simulink model "powerwindow03"  (R2019b)
settings: Solver=ode23tb  StartTime=0.0  StopTime=inf  FixedStep=1e-4  RelTol=1e-2  EnableMultiTasking=on
libraries: mblibv1 x19, powerlib x15, simulink x4, vrlib x1
(part 1 of 2)
settings Model: FPTRunName=Active  ExtModeAutoUpdateStatusClock=off  Creator=The MathWorks Inc.  LastModifiedBy=bhisma
settings DataIOCC: LimitDataPoints=on  SaveFormat=Array  SignalLoggingSaveFormat=ModelDataLogs  ReturnWorkspaceOutputs=off  SignalLoggingName=sigsOut
settings OptimizationCC: BooleanDataType=off  ExpressionDepthLimit=2147483647  InitFltsAndDblsToZero=on  LifeSpan=inf
settings DebuggingCC: SaveWithParameterizedLinksMsg=none  UnderspecifiedInitializationDetection=Classic  MergeDetectMultiDrivingBlocksExec=none  CheckExecutionContextPreStartOutputMsg=on  CheckExecutionContextRuntimeOutputMsg=on  SignalResolutionControl=TryResolveAllWithWarning  MultiTaskDSMMsg=warning  MultiTaskCondExecSysMsg=none  FcnCallInpInsideContextMsg=warning  StateNameClashWarn=warning  SFUnexpectedBacktrackingDiag=warning  SFNoUnconditionalDefaultTransitionDiag=warning  SFExecutionAtInitializationDiag=none  ArithmeticOperatorsInVariantConditions=warning
settings HardwareCC: ProdBitPerPointer=32  ProdBitPerSizeT=32  ProdBitPerPtrDiffT=32  ProdLargestAtomicFloat=None  ProdIntDivRoundTo=Undefined  ProdEndianess=Unspecified  ProdWordSize=32  ProdHWDeviceType=32-bit Generic
settings ModelReferenceCC: PropagateSignalLabelsOutOfModel=off
settings SFSimCC: SimUseLocalCustomCode=off  SimParseCustomCode=off  CustomCodeUndefinedFunction=UseInterfaceOnly
settings RTWCC: RTWUseLocalCustomCode=off
settings CodeAppCC: StateflowObjectComments=on
settings GRTTargetCC: TargetFcnLib=ansi_tfl_tmw.mat  TargetLangStandard=C89/C90 (ANSI)  GeneratePreprocessorConditionals=Disable all  CombineOutputUpdateFcns=off  GRTInterface=on
settings ConfigComp: CovMetricSettings=dw  CovHtmlReporting=on  CovSaveCumulativeToWorkspaceVar=on  CovSaveSingleToWorkspaceVar=on  CovExternalEMLEnable=off
settings SimscapeCC: SimscapeNormalizeSystem=off
settings SimMechanicsCC: WarnOnRedundantConstraints=off  VisOnUpdateDiagram=on

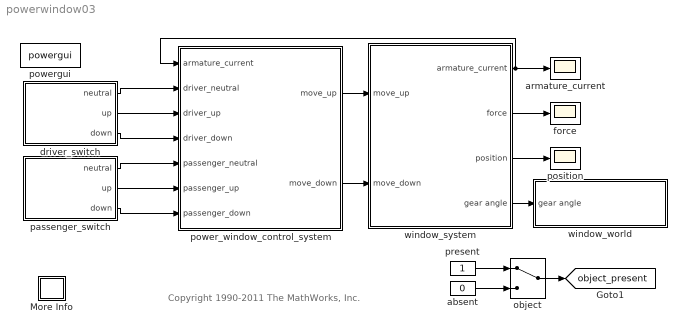
== system powerwindow03 ==
  note: Copyright 1990-2011 The MathWorks, Inc.
  More Info : Subsystem
      settings: OpenFcn=showdemo(bdroot(gcb))
      mask Display: disp('?')
  absent : Constant  Value=0
  armature_current : Scope
  driver_switch : Subsystem
  force : Scope
  object : ManualSwitch
  passenger_switch : Subsystem
  position : Scope
  power_window_control_system : Subsystem
  powergui : powerlib/powergui  SimulationMode=Continuous  SampleTime=0  frequency=60  Iterations=50  frequencyindice=0  Pbase=100e6  ErrMax=1e-4  UnitsV=kV  UnitsW=MW  buscounter=0  FunctionMessages=off  echomessages=off  EnableUseOfTLC=off  CurrentSourceSwitches=off  DisableSnubberDevices=off  DisableRonSwitches=off  DisableVfSwitches=off  DisplayEquations=off  AutomaticDiscreteSolvers=off  SolverType=Tustin  Interpol=off  ExternalGateDelay=off  methode=off  Ts=0  x0status=blocks  SPID=off  SwTol=0  HookPort=off  NonlinearTolerance=1e-4  nMaxIteration=100  ContinueOnMaxIteration=off  RestoreLinks=warning  ResistiveCurrentMeasurement=off  Frange=[0:2:500]  Ylog=off  Xlog=on  ShowGrid=off  save=off  variable=ZData  structure=0  ZoomFFT=on  StartTime=0.0  cycles=1  DisplayStyle=1  fundamental=60  FreqAxis=off  MaxFrequency=1000  frequencyindicesteady=1  RmsSteady=1  display=off
      settings: SourceProductName=Simscape Electrical
  present : Constant
  window_system : Subsystem
  window_world : Subsystem
  tag scope: object_present=global
  wires:
  driver_switch/1(neutral) -> power_window_control_system/2(driver_neutral)
  driver_switch/2(up) -> power_window_control_system/3(driver_up)
  driver_switch/3(down) -> power_window_control_system/4(driver_down)
  passenger_switch/1(neutral) -> power_window_control_system/5(passenger_neutral)
  passenger_switch/2(up) -> power_window_control_system/6(passenger_up)
  passenger_switch/3(down) -> power_window_control_system/7(passenger_down)
  power_window_control_system/1(move_up) -> window_system/1(move_up)
  power_window_control_system/2(move_down) -> window_system/2(move_down)
  window_system/1(armature_current) -> armature_current/1, power_window_control_system/1(armature_current)
  window_system/2(force) -> force/1
  window_system/3(position) -> position/1
  present/1 -> object/1
  absent/1 -> object/2
  object/1 -> [object_present]
  window_system/4(gear angle) -> window_world/1(gear angle)

== system powerwindow03/More Info ==

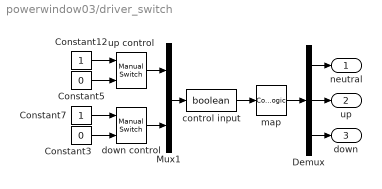
== system powerwindow03/driver_switch ==
  Constant12 : Constant
  Constant3 : Constant  Value=0
  Constant5 : Constant  Value=0
  Constant7 : Constant
  Demux : Demux  Outputs=3
  Mux1 : Mux  Inputs=2
  control input : DataTypeConversion  OutDataTypeStr=boolean  SaturateOnIntegerOverflow=on  RndMeth=Zero
  down control : simulink/Signal Routing/Manual Switch  sw=0  action=0  varsize=off
      settings: SourceProductName=Simulink  SourceProductBaseCode=SL
  map : CombinatorialLogic  TruthTable=[1 0 0;0 0 1;0 1 0;1 0 0]
  up control : simulink/Signal Routing/Manual Switch  sw=1  action=0  varsize=off
      settings: SourceProductName=Simulink  SourceProductBaseCode=SL
  neutral : Outport
  up : Outport  Port=2
  down : Outport  Port=3
  wires:
  control input/1 -> map/1
  Constant12/1 -> up control/1
  Constant5/1 -> up control/2
  Constant7/1 -> down control/1
  Constant3/1 -> down control/2
  down control/1 -> Mux1/2
  Mux1/1 -> control input/1
  up control/1 -> Mux1/1
  map/1 -> Demux/1
  Demux/1 -> neutral/1
  Demux/2 -> up/1
  Demux/3 -> down/1

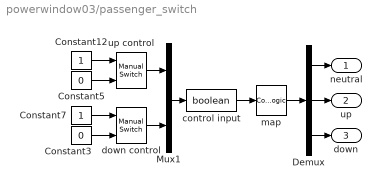
== system powerwindow03/passenger_switch ==
  Constant12 : Constant
  Constant3 : Constant  Value=0
  Constant5 : Constant  Value=0
  Constant7 : Constant
  Demux : Demux  Outputs=3
  Mux1 : Mux  Inputs=2
  control input : DataTypeConversion  OutDataTypeStr=boolean  SaturateOnIntegerOverflow=on  RndMeth=Zero
  down control : simulink/Signal Routing/Manual Switch  sw=0  action=0  varsize=off
      settings: SourceProductName=Simulink  SourceProductBaseCode=SL
  map : CombinatorialLogic  TruthTable=[1 0 0;0 0 1;0 1 0;1 0 0]
  up control : simulink/Signal Routing/Manual Switch  sw=0  action=0  varsize=off
      settings: SourceProductName=Simulink  SourceProductBaseCode=SL
  neutral : Outport
  up : Outport  Port=2
  down : Outport  Port=3
  wires:
  Demux/3 -> down/1
  Demux/2 -> up/1
  Demux/1 -> neutral/1
  map/1 -> Demux/1
  up control/1 -> Mux1/1
  Mux1/1 -> control input/1
  down control/1 -> Mux1/2
  Constant3/1 -> down control/2
  Constant7/1 -> down control/1
  Constant5/1 -> up control/2
  Constant12/1 -> up control/1
  control input/1 -> map/1

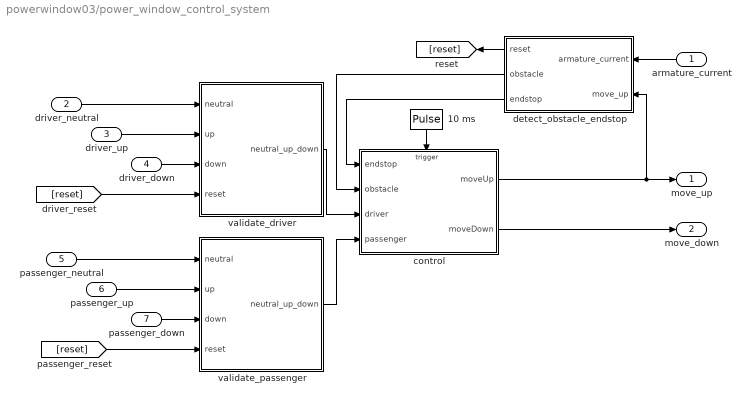
== system powerwindow03/power_window_control_system ==
  armature_current : Inport
  driver_neutral : Inport  Port=2
  driver_up : Inport  Port=3
  driver_down : Inport  Port=4
  passenger_neutral : Inport  Port=5
  passenger_up : Inport  Port=6
  passenger_down : Inport  Port=7
  10 ms : DiscretePulseGenerator  SampleTime=10e-3
  control : Stateflow chart  TreatAsAtomicUnit=on
  detect_obstacle_endstop : Subsystem
  validate_driver : Subsystem
  validate_passenger : Subsystem
  move_up : Outport
  move_down : Outport  Port=2
  wires:
  detect_obstacle_endstop/2(obstacle) -> control/2(obstacle)
  detect_obstacle_endstop/3(endstop) -> control/1(endstop)
  detect_obstacle_endstop/1(reset) -> [reset]
  armature_current/1 -> detect_obstacle_endstop/1(armature_current)
  10 ms/1 -> control/Trigger
  control/1(moveUp) -> detect_obstacle_endstop/2(move_up), move_up/1
  control/2(moveDown) -> move_down/1
  driver_neutral/1 -> validate_driver/1(neutral)
  driver_up/1 -> validate_driver/2(up)
  driver_down/1 -> validate_driver/3(down)
  [reset] -> validate_driver/4(reset)
  passenger_neutral/1 -> validate_passenger/1(neutral)
  passenger_up/1 -> validate_passenger/2(up)
  passenger_down/1 -> validate_passenger/3(down)
  [reset] -> validate_passenger/4(reset)
  validate_driver/1(neutral_up_down) -> control/3(driver)
  validate_passenger/1(neutral_up_down) -> control/4(passenger)

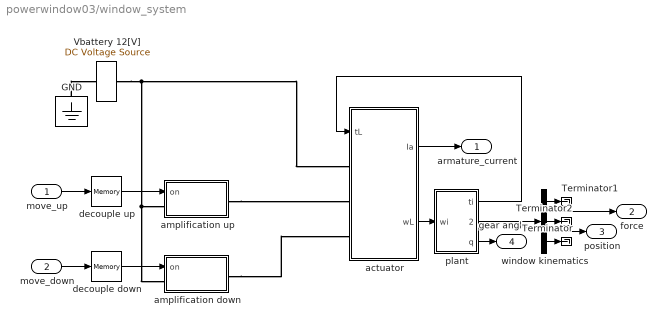
== system powerwindow03/window_system ==
  move_up : Inport
  move_down : Inport  Port=2
  GND : powerlib/Elements/Ground  LConnTagsString=a
      settings: SourceProductName=Simscape Electrical
  Terminator : Terminator
  Terminator1 : Terminator
  Terminator2 : Terminator
  Vbattery 12[V] : powerlib/Electrical Sources/DC Voltage Source  Amplitude=12  Measurements=None
      settings: SourceProductName=Simscape Electrical
  actuator : Subsystem
  amplification down : Subsystem
  amplification up : Subsystem
  decouple down : Memory
  decouple up : Memory
  plant : Subsystem
  window kinematics : Demux  Outputs=[1,1,2,1,4]
  armature_current : Outport
  force : Outport  Port=2
  position : Outport  Port=3
  gear angle : Outport  Port=4
  wires:
  decouple down/1 -> amplification down/1(on)
  decouple up/1 -> amplification up/1(on)
  plant/3(q) -> gear angle/1
  actuator/2(wL) -> plant/1(wi)
  plant/2("F, x, v") -> window kinematics/1
  actuator/1(Ia) -> armature_current/1
  move_up/1 -> decouple up/1
  move_down/1 -> decouple down/1
  window kinematics/2 -> force/1
  window kinematics/1 -> Terminator1/1
  window kinematics/4 -> position/1
  window kinematics/5 -> Terminator/1
  window kinematics/3 -> Terminator2/1
  plant/1(ti) -> actuator/1(tL)
  connections:
  GND/LConn1 -- Vbattery 12[V]/LConn1
  amplification up/RConn1 -- actuator/LConn2
  amplification down/RConn1 -- actuator/LConn3
  Vbattery 12[V]/RConn1 -- amplification down/LConn1 -- amplification up/LConn1 -- actuator/LConn1

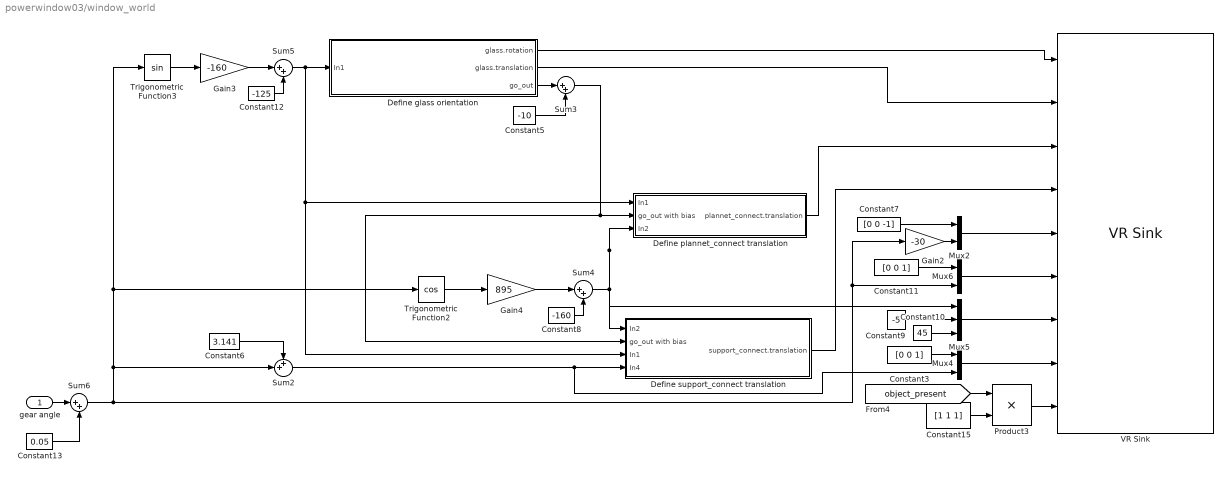
== system powerwindow03/window_world ==
  gear angle : Inport
  Constant10 : Constant  Value=45
  Constant11 : Constant  Value=[0 0 1]
  Constant12 : Constant  Value=-125
  Constant13 : Constant  Value=0.05
  Constant15 : Constant  Value=[1 1 1]
  Constant3 : Constant  Value=[0 0 1]
  Constant5 : Constant  Value=-10
  Constant6 : Constant  Value=3.141
  Constant7 : Constant  Value=[0 0 -1]
  Constant8 : Constant  Value=-160
  Constant9 : Constant  Value=-5
  Define glass orientation : Subsystem
  Define plannet_connect translation : Subsystem
  Define support_connect translation : Subsystem
  Gain2 : Gain  Gain=-30  SaturateOnIntegerOverflow=on  OutDataTypeStr=Inherit: Same as input  ParamDataTypeStr=Inherit: Same as input
  Gain3 : Gain  Gain=-160  SaturateOnIntegerOverflow=on  OutDataTypeStr=Inherit: Same as input  ParamDataTypeStr=Inherit: Same as input
  Gain4 : Gain  Gain=895  SaturateOnIntegerOverflow=on  OutDataTypeStr=Inherit: Same as input  ParamDataTypeStr=Inherit: Same as input
  Mux2 : Mux  Inputs=2
  Mux4 : Mux  Inputs=2
  Mux5 : Mux  Inputs=3
  Mux6 : Mux  Inputs=2
  Product3 : Product  SaturateOnIntegerOverflow=on  InputSameDT=on  OutDataTypeStr=Inherit: Same as first input
  Sum2 : Sum  Inputs=++|  SaturateOnIntegerOverflow=on  InputSameDT=on  OutDataTypeStr=Inherit: Same as first input
  Sum{3..6} (4 alike) : Sum  Inputs=|++  SaturateOnIntegerOverflow=on  InputSameDT=on  OutDataTypeStr=Inherit: Same as first input
  Trigonometric Function2 : Trigonometry  Operator=cos
  Trigonometric Function3 : Trigonometry
  VR Sink : vrlib/VR Sink  SampleTime=0.1  ViewEnable=on  RemoteChange=off  RemoteView=on  FieldsWritten=glass.rotation.4.1.1.double#glass.translation.3.1.1.double#plannet_connect.translation.3.1.1.double#support_connect.translation.3.1.1.double#worm.rotation.4.1.1.double#planetROT.rotation.4.1.1.double#support.translation.3.1.1.double#supportROT.rotation.4.1.1.double#balloon.scale.3.1.1.double  WorldFileName=pw_mech_window_world.wrl  WorldDescription=VR Power Window Model  AutoView=on  VideoDimensions=[]  AllowVariableSize=off  FigureProperties="{'Position', 'Name', 'Viewpoint', 'CameraBound', 'CameraDirection', 'CameraPosition', 'CameraUpVector', 'ZoomFactor', 'Antialiasing', 'Headlight', 'Lighting', 'NavPanel', 'StatusBar', 'ToolBar', 'Textures', 'Transparency', 'Wireframe', 'NavZones', 'NavMode', 'NavSpeed', 'Record2DCompressMethod', 'Record2DCompressQuality', 'Record2D', 'Record2DFileName', 'Record2DFPS'; [3.3000000000000000e+01   5.5200000000000000e+02   5.7600000000000000e+02   3.8000000000000000e+02], 'VR Power Window Model', 'Main View', 'on', [0.0000000000000000e+00   0.0000000000000000e+00  -1.0000000000000000e+00], [0.0000000000000000e+00   0.0000000000000000e+00   0.0000000000000000e+00], [0.0000000000000000e+00   1.0000000000000000e+00   0.0000000000000000e+00], [1.0000000000000000e+00], 'off', 'on', 'on', 'halfbar', 'on', 'on', 'on', 'on', 'off', 'off', 'examine', 'normal', 'auto', [7.5000000000000000e+01], 'off', '%f_anim_%n.avi', [1.5000000000000000e+01]}"
      settings: SourceProductName=Simulink
  wires:
  Constant5/1 -> Sum3/2
  Constant7/1 -> Mux2/1
  Gain2/1 -> Mux2/2
  Gain3/1 -> Sum5/1
  Constant12/1 -> Sum5/2
  Constant11/1 -> Mux6/1
  Trigonometric Function3/1 -> Gain3/1
  Constant8/1 -> Sum4/2
  Gain4/1 -> Sum4/1
  Trigonometric Function2/1 -> Gain4/1
  Constant10/1 -> Mux5/3
  Constant9/1 -> Mux5/2
  Sum2/1 -> Define support_connect translation/4(In4), Mux4/2
  Constant3/1 -> Mux4/1
  gear angle/1 -> Sum6/1
  Constant13/1 -> Sum6/2
  Constant15/1 -> Product3/2
  [object_present] -> Product3/1
  Define glass orientation/3(go_out) -> Sum3/1
  Sum6/1 -> Mux6/2, Gain2/1, Sum2/2, Trigonometric Function3/1, Trigonometric Function2/1
  Sum3/1 -> Define support_connect translation/2(go_out with bias), Define plannet_connect translation/2(go_out with bias)
  Sum5/1 -> Define plannet_connect translation/1(In1), Define support_connect translation/3(In1), Define glass orientation/1(In1)
  Sum4/1 -> Mux5/1, Define plannet_connect translation/3(In2), Define support_connect translation/1(In2)
  Constant6/1 -> Sum2/1
  Define glass orientation/1(glass.rotation) -> VR Sink/1
  Define glass orientation/2(glass.translation) -> VR Sink/2
  Define plannet_connect translation/1(plannet_connect.translation) -> VR Sink/3
  Mux2/1 -> VR Sink/5
  Mux6/1 -> VR Sink/6
  Mux5/1 -> VR Sink/7
  Define support_connect translation/1(support_connect.translation) -> VR Sink/4
  Mux4/1 -> VR Sink/8
  Product3/1 -> VR Sink/9

== system powerwindow03/power_window_control_system/detect_obstacle_endstop ==
  armature_current : Inport
  move_up : Inport  Port=2
  detect_endstop : Subsystem
  detect_obstacle : Subsystem
  either : Logic  Operator=OR
  process_current : Subsystem
  reset : Outport
  obstacle : Outport  Port=2
  endstop : Outport  Port=3
  wires:
  armature_current/1 -> process_current/1(raw_current)
  detect_obstacle/1(obstacle) -> either/1, obstacle/1
  detect_endstop/1(endstop) -> endstop/1, either/2
  either/1 -> reset/1
  move_up/1 -> detect_obstacle/1(move_up)
  process_current/1(processed_current) -> detect_obstacle/2(armature_current), detect_endstop/1(armature_current)

== system powerwindow03/power_window_control_system/validate_driver ==
  neutral : Inport
  up : Inport  Port=2
  down : Inport  Port=3
  reset : Inport  Port=4
  Mux : Mux  Inputs=3
  check_down : Subsystem
  check_up : Subsystem
  mutually_exclusive : Subsystem
  neutral_up_down : Outport
  wires:
  Mux/1 -> neutral_up_down/1
  reset/1 -> [reset]
  [reset] -> check_down/2(reset)
  [reset] -> check_up/2(reset)
  check_up/1(checked_action) -> mutually_exclusive/2(up)
  neutral/1 -> mutually_exclusive/1(neutral)
  up/1 -> check_up/1(action)
  down/1 -> check_down/1(action)
  mutually_exclusive/1(validated_neutral) -> Mux/1
  mutually_exclusive/2(validated_up) -> Mux/2
  mutually_exclusive/3(validated_down) -> Mux/3
  check_down/1(checked_action) -> mutually_exclusive/3(down)

== system powerwindow03/power_window_control_system/validate_passenger ==
  neutral : Inport
  up : Inport  Port=2
  down : Inport  Port=3
  reset : Inport  Port=4
  Mux : Mux  Inputs=3
  check_down : Subsystem
  check_up : Subsystem
  mutually_exclusive : Subsystem
  neutral_up_down : Outport
  wires:
  Mux/1 -> neutral_up_down/1
  reset/1 -> [reset]
  [reset] -> check_down/2(reset)
  [reset] -> check_up/2(reset)
  check_up/1(checked_action) -> mutually_exclusive/2(up)
  neutral/1 -> mutually_exclusive/1(neutral)
  up/1 -> check_up/1(action)
  down/1 -> check_down/1(action)
  mutually_exclusive/1(validated_neutral) -> Mux/1
  mutually_exclusive/2(validated_up) -> Mux/2
  mutually_exclusive/3(validated_down) -> Mux/3
  check_down/1(checked_action) -> mutually_exclusive/3(down)

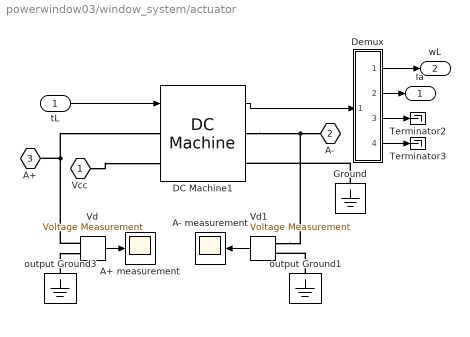
== system powerwindow03/window_system/actuator ==
  tL : Inport
  A+ measurement : Scope
  A- measurement : Scope
  DC Machine1 : powerlib/Machines/DC Machine  PresetModel=No  MechanicalLoad=Torque TL  FieldType=Wound  ShowDetailedParameters=on  RLa="[0.15  0.036]"  RLf=[1.5 3]  Laf=1  MachineConstant=Torque constant (N.m/A)  Ke=1.8  Kt=1.8  J=0.085  Bm=5  Tf=0  w0=0  Ifinit=8  TsPowergui=0  TsBlock=-1
      settings: SourceProductName=Simscape Electrical
  Demux : Subsystem
  Ground : powerlib/Elements/Ground  LConnTagsString=a
      settings: SourceProductName=Simscape Electrical
  Terminator2 : Terminator
  Terminator3 : Terminator
  Vd : powerlib/Measurements/Voltage Measurement  PhasorSimulation=off  OutputType=Magnitude  PSBequivalent=0
      settings: SourceProductName=Simscape Electrical
  Vd1 : powerlib/Measurements/Voltage Measurement  PhasorSimulation=off  OutputType=Magnitude  PSBequivalent=0
      settings: SourceProductName=Simscape Electrical
  output Ground1 : powerlib/Elements/Ground  LConnTagsString=a
      settings: SourceProductName=Simscape Electrical
  output Ground3 : powerlib/Elements/Ground  LConnTagsString=a
      settings: SourceProductName=Simscape Electrical
  Vcc : PMIOPort  Side=Left
  A- : PMIOPort  Port=2  Side=Left
  A+ : PMIOPort  Port=3  Side=Left
  Ia : Outport
  wL : Outport  Port=2
  wires:
  Demux/4(Te) -> Terminator3/1
  Demux/3(If) -> Terminator2/1
  DC Machine1/1 -> Demux/1(m)
  Demux/2(Ia) -> Ia/1
  Vd/1 -> A+ measurement/1
  Vd1/1 -> A- measurement/1
  Demux/1(wm) -> wL/1
  tL/1 -> DC Machine1/1
  connections:
  output Ground3/LConn1 -- Vd/LConn2
  output Ground1/LConn1 -- Vd1/LConn2
  Ground/LConn1 -- DC Machine1/RConn2
  Vd1/LConn1 -- A-/RConn1 -- DC Machine1/RConn1
  Vcc/RConn1 -- DC Machine1/LConn2
  Vd/LConn1 -- A+/RConn1 -- DC Machine1/LConn1

== system powerwindow03/window_system/amplification down ==
  on : Inport
  Logical Operator : Logic  Operator=NOT
  Terminator1 : Terminator
  Terminator2 : Terminator
  output Ground1 : powerlib/Elements/Ground  LConnTagsString=a
      settings: SourceProductName=Simscape Electrical
  up switch : powerlib/Power Electronics/Ideal Switch  Ron=0.01  Lon=0  IC=0  Rs=1000000  Cs=inf  Measurements=on
      settings: SourceProductName=Simscape Electrical
  up switch1 : powerlib/Power Electronics/Ideal Switch  Ron=0.01  Lon=0  IC=0  Rs=1000000  Cs=inf  Measurements=on
      settings: SourceProductName=Simscape Electrical
  Vcc : PMIOPort  Side=Left
  pin : PMIOPort  Port=2  Side=Right
  wires:
  on/1 -> up switch/1, Logical Operator/1
  up switch/1 -> Terminator1/1
  up switch1/1 -> Terminator2/1
  Logical Operator/1 -> up switch1/1
  connections:
  Vcc/RConn1 -- up switch/LConn1
  up switch/RConn1 -- pin/RConn1 -- up switch1/RConn1
  up switch1/LConn1 -- output Ground1/LConn1

== system powerwindow03/window_system/amplification up ==
  on : Inport
  Logical Operator : Logic  Operator=NOT
  Terminator1 : Terminator
  Terminator2 : Terminator
  output Ground1 : powerlib/Elements/Ground  LConnTagsString=a
      settings: SourceProductName=Simscape Electrical
  up switch : powerlib/Power Electronics/Ideal Switch  Ron=0.01  Lon=0  IC=0  Rs=1000000  Cs=inf  Measurements=on
      settings: SourceProductName=Simscape Electrical
  up switch1 : powerlib/Power Electronics/Ideal Switch  Ron=0.01  Lon=0  IC=0  Rs=1000000  Cs=inf  Measurements=on
      settings: SourceProductName=Simscape Electrical
  Vcc : PMIOPort  Side=Left
  pin : PMIOPort  Port=2  Side=Right
  wires:
  on/1 -> up switch/1, Logical Operator/1
  up switch/1 -> Terminator1/1
  up switch1/1 -> Terminator2/1
  Logical Operator/1 -> up switch1/1
  connections:
  Vcc/RConn1 -- up switch/LConn1
  up switch1/LConn1 -- output Ground1/LConn1
  pin/RConn1 -- up switch/RConn1 -- up switch1/RConn1

== system powerwindow03/window_system/plant ==
  wi : Inport
  Demux1 : Demux  Outputs=[4, 1, 2, 1, 1]
  Terminator : Terminator
  Terminator1 : Terminator
  Terminator2 : Terminator
  object : Subsystem
  window : Subsystem
  ti : Outport
  "F, x, v" : Outport  Port=2
  q : Outport  Port=3
  wires:
  window/2(ti) -> ti/1
  wi/1 -> window/1(wi)
  object/1(torque) -> window/2(Fx)
  window/3(q) -> q/1
  Demux1/4 -> object/2(velocity)
  Demux1/2 -> object/1(position)
  Demux1/1 -> Terminator/1
  Demux1/3 -> Terminator1/1
  Demux1/5 -> Terminator2/1
  window/1(F,d,v) -> Demux1/1, "F, x, v"/1

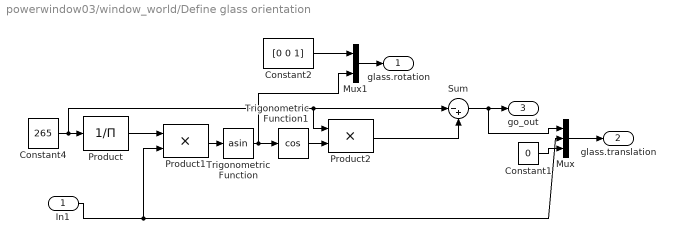
== system powerwindow03/window_world/Define glass orientation ==
  In1 : Inport
  Constant1 : Constant  Value=0
  Constant2 : Constant  Value=[0 0 1]
  Constant4 : Constant  Value=265
  Mux : Mux  Inputs=3
  Mux1 : Mux  Inputs=2
  Product : Product  Inputs=/  SaturateOnIntegerOverflow=on  InputSameDT=on  OutDataTypeStr=Inherit: Same as first input
  Product1 : Product  SaturateOnIntegerOverflow=on  InputSameDT=on  OutDataTypeStr=Inherit: Same as first input
  Product2 : Product  SaturateOnIntegerOverflow=on  InputSameDT=on  OutDataTypeStr=Inherit: Same as first input
  Sum : Sum  Inputs=|-+  SaturateOnIntegerOverflow=on  InputSameDT=on  OutDataTypeStr=Inherit: Same as first input
  Trigonometric Function : Trigonometry  Operator=asin
  Trigonometric Function1 : Trigonometry  Operator=cos
  glass.rotation : Outport
  glass.translation : Outport  Port=2
  go_out : Outport  Port=3
  wires:
  Mux/1 -> glass.translation/1
  Mux1/1 -> glass.rotation/1
  In1/1 -> Product1/2, Mux/2
  Constant1/1 -> Mux/3
  Constant2/1 -> Mux1/1
  Constant4/1 -> Product/1, Product2/1, Sum/1
  Product/1 -> Product1/1
  Product1/1 -> Trigonometric Function/1
  Trigonometric Function/1 -> Trigonometric Function1/1, Mux1/2
  Trigonometric Function1/1 -> Product2/2
  Product2/1 -> Sum/2
  Sum/1 -> go_out/1, Mux/1

== system powerwindow03/window_world/Define plannet_connect translation ==
  In1 : Inport
  go_out with bias : Inport  Port=2
  In2 : Inport  Port=3
  Gain1 : Gain  Gain=0.265  SaturateOnIntegerOverflow=on  OutDataTypeStr=Inherit: Same as input  ParamDataTypeStr=Inherit: Same as input
  Mux3 : Mux  Inputs=3
  plannet_connect.translation : Outport
  wires:
  Mux3/1 -> plannet_connect.translation/1
  In2/1 -> Gain1/1
  In1/1 -> Mux3/2
  go_out with bias/1 -> Mux3/1
  Gain1/1 -> Mux3/3

== system powerwindow03/window_world/Define support_connect translation ==
  In2 : Inport
  go_out with bias : Inport  Port=2
  In1 : Inport  Port=3
  In4 : Inport  Port=4
  Constant14 : Constant  Value=305
  Gain5 : Gain  Gain=1000  SaturateOnIntegerOverflow=on  OutDataTypeStr=Inherit: Same as input  ParamDataTypeStr=Inherit: Same as input
  Gain6 : Gain  Gain=0.265  SaturateOnIntegerOverflow=on  OutDataTypeStr=Inherit: Same as input  ParamDataTypeStr=Inherit: Same as input
  Mux7 : Mux  Inputs=3
  Sum1 : Sum  Inputs=+++  SaturateOnIntegerOverflow=on  InputSameDT=on  OutDataTypeStr=Inherit: Same as first input
  Trigonometric Function4 : Trigonometry  Operator=cos
  support_connect.translation : Outport
  wires:
  Mux7/1 -> support_connect.translation/1
  In4/1 -> Trigonometric Function4/1
  In2/1 -> Sum1/1
  In1/1 -> Mux7/2
  go_out with bias/1 -> Mux7/1
  Trigonometric Function4/1 -> Gain5/1
  Gain5/1 -> Sum1/2
  Sum1/1 -> Gain6/1
  Gain6/1 -> Mux7/3
  Constant14/1 -> Sum1/3

== system powerwindow03/power_window_control_system/detect_obstacle_endstop/detect_endstop ==
  armature_current : Inport
  Constant6 : Constant  Value=15
  current_limit : RelationalOperator  Operator=>  RndMeth=Nearest  InputSameDT=on
  passenger control : DataTypeConversion  OutDataTypeStr=boolean  SaturateOnIntegerOverflow=on  RndMeth=Zero
  endstop : Outport
  wires:
  passenger control/1 -> endstop/1
  current_limit/1 -> passenger control/1
  armature_current/1 -> current_limit/1
  Constant6/1 -> current_limit/2

== system powerwindow03/power_window_control_system/detect_obstacle_endstop/detect_obstacle ==
  move_up : Inport
  armature_current : Inport  Port=2
  10 ms1 : DiscretePulseGenerator  SampleTime=10e-3
  Constant1 : Constant  Value=1.2
  Product : Product  SaturateOnIntegerOverflow=on  InputSameDT=on  OutDataTypeStr=Inherit: Same as first input
  break dependency : UnitDelay  SampleTime=0.01  HasFrameUpgradeWarning=on
  delay_detection : Stateflow chart  TreatAsAtomicUnit=on
  object : RelationalOperator  Operator=>  RndMeth=Nearest  InputSameDT=on
  passenger control : DataTypeConversion  OutDataTypeStr=boolean  SaturateOnIntegerOverflow=on  RndMeth=Zero
  obstacle : Outport
  wires:
  passenger control/1 -> obstacle/1
  break dependency/1 -> delay_detection/1(move_up)
  10 ms1/1 -> delay_detection/Trigger
  Product/1 -> passenger control/1
  move_up/1 -> break dependency/1
  armature_current/1 -> object/1
  delay_detection/1(" detect") -> Product/2
  object/1 -> Product/1
  Constant1/1 -> object/2

== system powerwindow03/power_window_control_system/detect_obstacle_endstop/process_current ==
  raw_current : Inport
  Abs : Abs  SaturateOnIntegerOverflow=on
  processed_current : Outport
  wires:
  raw_current/1 -> Abs/1
  Abs/1 -> processed_current/1

== system powerwindow03/power_window_control_system/validate_driver/check_down ==
  action : Inport
  reset : Inport  Port=2
  allow_action : Logic
  overrule : Logic  Operator=NOT
  checked_action : Outport
  wires:
  reset/1 -> overrule/1
  allow_action/1 -> checked_action/1
  action/1 -> allow_action/1
  overrule/1 -> allow_action/2

== system powerwindow03/power_window_control_system/validate_driver/check_up ==
  action : Inport
  reset : Inport  Port=2
  allow_action : Logic
  overrule : Logic  Operator=NOT
  checked_action : Outport
  wires:
  overrule/1 -> allow_action/2
  action/1 -> allow_action/1
  allow_action/1 -> checked_action/1
  reset/1 -> overrule/1

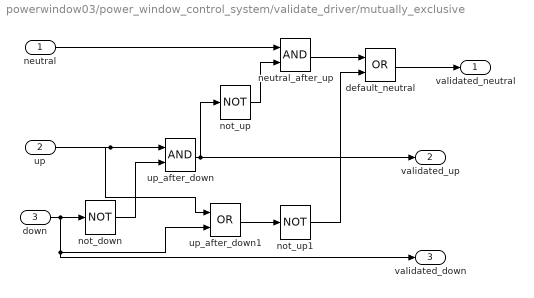
== system powerwindow03/power_window_control_system/validate_driver/mutually_exclusive ==
  neutral : Inport
  up : Inport  Port=2
  down : Inport  Port=3
  default_neutral : Logic  Operator=OR
  neutral_after_up : Logic
  not_down : Logic  Operator=NOT
  not_up : Logic  Operator=NOT
  not_up1 : Logic  Operator=NOT
  up_after_down : Logic
  up_after_down1 : Logic  Operator=OR
  validated_neutral : Outport
  validated_up : Outport  Port=2
  validated_down : Outport  Port=3
  wires:
  not_down/1 -> up_after_down/2
  up_after_down/1 -> not_up/1, validated_up/1
  not_up/1 -> neutral_after_up/2
  down/1 -> not_down/1, up_after_down1/2, validated_down/1
  neutral/1 -> neutral_after_up/1
  up/1 -> up_after_down/1, up_after_down1/1
  up_after_down1/1 -> not_up1/1
  neutral_after_up/1 -> default_neutral/1
  default_neutral/1 -> validated_neutral/1
  not_up1/1 -> default_neutral/2

== system powerwindow03/power_window_control_system/validate_passenger/check_down ==
  action : Inport
  reset : Inport  Port=2
  allow_action : Logic
  overrule : Logic  Operator=NOT
  checked_action : Outport
  wires:
  reset/1 -> overrule/1
  allow_action/1 -> checked_action/1
  action/1 -> allow_action/1
  overrule/1 -> allow_action/2

== system powerwindow03/power_window_control_system/validate_passenger/check_up ==
  action : Inport
  reset : Inport  Port=2
  allow_action : Logic
  overrule : Logic  Operator=NOT
  checked_action : Outport
  wires:
  overrule/1 -> allow_action/2
  action/1 -> allow_action/1
  allow_action/1 -> checked_action/1
  reset/1 -> overrule/1

== system powerwindow03/power_window_control_system/validate_passenger/mutually_exclusive ==
  neutral : Inport
  up : Inport  Port=2
  down : Inport  Port=3
  default_neutral : Logic  Operator=OR
  neutral_after_up : Logic
  not_down : Logic  Operator=NOT
  not_up : Logic  Operator=NOT
  not_up1 : Logic  Operator=NOT
  up_after_down : Logic
  up_after_down1 : Logic  Operator=OR
  validated_neutral : Outport
  validated_up : Outport  Port=2
  validated_down : Outport  Port=3
  wires:
  not_down/1 -> up_after_down/2
  up_after_down/1 -> not_up/1, validated_up/1
  not_up/1 -> neutral_after_up/2
  down/1 -> not_down/1, up_after_down1/2, validated_down/1
  neutral/1 -> neutral_after_up/1
  up/1 -> up_after_down/1, up_after_down1/1
  up_after_down1/1 -> not_up1/1
  neutral_after_up/1 -> default_neutral/1
  default_neutral/1 -> validated_neutral/1
  not_up1/1 -> default_neutral/2

== system powerwindow03/window_system/actuator/Demux ==
  m : Inport
  Demux : Demux
  wm : Outport
  Ia : Outport  Port=2
  If : Outport  Port=3
  Te : Outport  Port=4
  wires:
  Demux/4 -> Te/1
  Demux/3 -> If/1
  m/1 -> Demux/1
  Demux/2 -> Ia/1
  Demux/1 -> wm/1

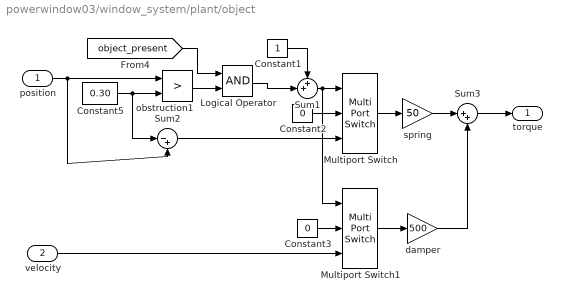
== system powerwindow03/window_system/plant/object ==
  position : Inport
  velocity : Inport  Port=2
  Constant1 : Constant
  Constant2 : Constant  Value=0
  Constant3 : Constant  Value=0
  Constant5 : Constant  Value=0.30
  Logical Operator : Logic
  Multiport Switch : MultiPortSwitch  Inputs=2  InputSameDT=on
  Multiport Switch1 : MultiPortSwitch  Inputs=2  InputSameDT=on
  Sum1 : Sum  Inputs=++|  SaturateOnIntegerOverflow=on  InputSameDT=on  OutDataTypeStr=Inherit: Same as first input
  Sum2 : Sum  Inputs=|-+  SaturateOnIntegerOverflow=on  InputSameDT=on  OutDataTypeStr=Inherit: Same as first input
  Sum3 : Sum  Inputs=|++  SaturateOnIntegerOverflow=on  InputSameDT=on  OutDataTypeStr=Inherit: Same as first input
  damper : Gain  Gain=500  SaturateOnIntegerOverflow=on  OutDataTypeStr=Inherit: Same as input  ParamDataTypeStr=Inherit: Same as input
  obstruction1 : RelationalOperator  Operator=>  RndMeth=Nearest  InputSameDT=on
  spring : Gain  Gain=50  SaturateOnIntegerOverflow=on  OutDataTypeStr=Inherit: Same as input  ParamDataTypeStr=Inherit: Same as input
  torque : Outport
  wires:
  [object_present] -> Logical Operator/1
  Logical Operator/1 -> Sum1/2
  obstruction1/1 -> Logical Operator/2
  Multiport Switch1/1 -> damper/1
  velocity/1 -> Multiport Switch1/3
  Constant3/1 -> Multiport Switch1/2
  Multiport Switch/1 -> spring/1
  position/1 -> Sum2/2, obstruction1/1
  Constant1/1 -> Sum1/1
  Sum2/1 -> Multiport Switch/3
  Constant2/1 -> Multiport Switch/2
  Sum1/1 -> Multiport Switch1/1, Multiport Switch/1
  Constant5/1 -> Sum2/1, obstruction1/2
  damper/1 -> Sum3/2
  Sum3/1 -> torque/1
  spring/1 -> Sum3/1

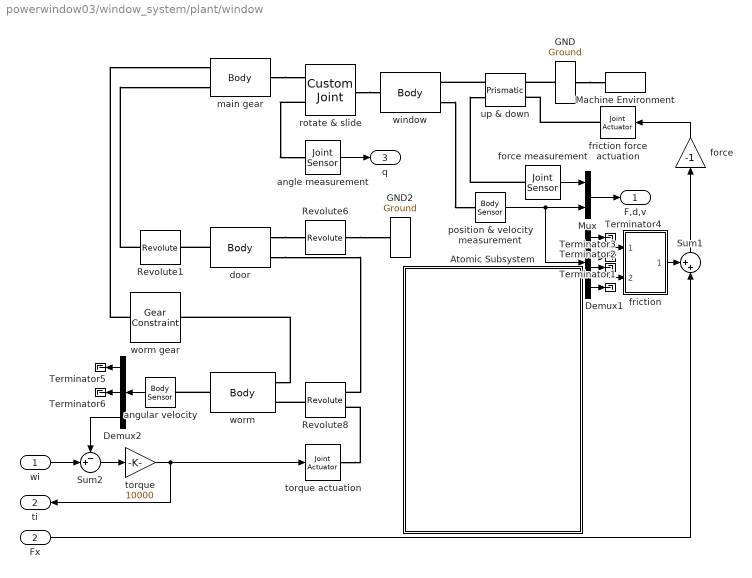
== system powerwindow03/window_system/plant/window ==
  wi : Inport
  Fx : Inport  Port=2
  Atomic Subsystem : Subsystem  TreatAsAtomicUnit=on
      mask Display: image(imread([matlabroot,'/toolbox/simulink/simdemos/automotive/html/pw_window1c.jpg']))
  Demux1 : Demux  Outputs=6
  Demux2 : Demux  Outputs=3
  GND : mblibv1/Bodies/Ground  UpdateFromCAD=off  LeftPortType=env  RightPortType=workingframe  PhysicalDomain=Mechanical  DialogClass=GroundBlock  CoordPosition=[10 0 0]  CoordPositionUnits=cm  StateVectorMgrId=0  MachineId=[1 0]  ShowEnvPort=on
      settings: SourceProductName=Simscape Multibody  SourceProductBaseCode=MS
  GND2 : mblibv1/Bodies/Ground  UpdateFromCAD=off  LeftPortType=env  RightPortType=workingframe  PhysicalDomain=Mechanical  DialogClass=GroundBlock  CoordPosition=[0 0 0]  CoordPositionUnits=m  StateVectorMgrId=-1  MachineId=[0 0]  ShowEnvPort=off
      settings: SourceProductName=Simscape Multibody  SourceProductBaseCode=MS
  Machine Environment : mblibv1/Bodies/Machine Environment  Tag=Factory ground  PortType=env  PhysicalDomain=Mechanical  DialogTemplateClass=MECH.MachineEnvironment  SyncWhenCopied=off  Gravity=[0 0 0]  GravityUnits=m/s^2  GravityAsSignal=off  Dimensionality=3D Only  AnalysisType=Forward dynamics  LinearAssemblyTolerance=1e-3  LinearAssemblyToleranceUnits=m  AngularAssemblyTolerance=1e-3  AngularAssemblyToleranceUnits=rad  ConstraintSolverType=Stabilizing  ConstraintRelTolerance=1e-4  ConstraintAbsTolerance=1e-4  UseRobustSingularityHandling=off  RedundancyAnalysisToleranceType=Automatically select tolerance  RedundancyAnalysisTolerance=1e-14  StatePerturbationType=Fixed  PerturbationSize=1e-5  VisualizeMachine=on  BodyVisualizationType=Use model default body geometries  BodyColorSelMode=Use model default  DefaultBodyColor=[1 0 0]
      settings: SourceProductName=Simscape Multibody  SourceProductBaseCode=MS
  Mux : Mux  Inputs=2
  Revolute1 : mblibv1/Joints/Revolute  Tag=Factory generic  Description=Mechanical Blockset  LConnTagsString=__newl0  RConnTagsString=__newr0  UpdateFromCAD=off  NumSAPorts=0  CutJoint=off  MarkAsCut=off  Primitives=revolute  PrimitiveProps=R1$WORLD$[0 0 1]$revolute  DialogClass=JointBlock  R1Axis=[0 0 1]
      settings: SourceProductName=Simscape Multibody  SourceProductBaseCode=MS
  Revolute6 : mblibv1/Joints/Revolute  Tag=Factory generic  Description=Mechanical Blockset  LConnTagsString=__newl0  RConnTagsString=__newr0  UpdateFromCAD=off  NumSAPorts=0  CutJoint=off  MarkAsCut=off  Primitives=revolute  PrimitiveProps=R1$WORLD$[1 0 0]$revolute  DialogClass=JointBlock  R1Axis=[1 0 0]
      settings: SourceProductName=Simscape Multibody  SourceProductBaseCode=MS
  Revolute8 : mblibv1/Joints/Revolute  Tag=Factory generic  Description=Mechanical Blockset  LConnTagsString=__newl0|SA1  RConnTagsString=__newr0  UpdateFromCAD=off  NumSAPorts=1  CutJoint=off  MarkAsCut=off  Primitives=revolute  PrimitiveProps=R1$WORLD$[0 0 1]$revolute  DialogClass=JointBlock  R1Axis=[0 0 1]
      settings: SourceProductName=Simscape Multibody  SourceProductBaseCode=MS
  Sum1 : Sum  Inputs=++|  SaturateOnIntegerOverflow=on  InputSameDT=on  OutDataTypeStr=Inherit: Same as first input
  Sum2 : Sum  Inputs=-+|  SaturateOnIntegerOverflow=on  InputSameDT=on  OutDataTypeStr=Inherit: Same as first input
  Terminator{1..6} (6 alike) : Terminator
  angle measurement : mblibv1/Sensors &  Actuators/Joint Sensor  Description=Mechanical Blockset  UpdateFromCAD=off  PhysicalDomain=Mechanical  PortType=blob  Muxed=on  Pose=off  Angle=on  AngleUnits=rad  ArcVelocity=off  ArcVelocityUnits=deg/s  ArcAcceleration=off  ArcAccelerationUnits=deg/s^2  CoordPosition=off  CoordPositionUnits=m  Velocity=off  VelocityUnits=m/s  Acceleration=off  AccelerationUnits=m/s^2  Quaternion=on  QuaternionDT=off  QuaternionDDT=off  QuaternionUnits=off  OutputVector=[ 1 ]  ActiveIO=on  Width=1  DialogClass=MechanicalSensorBlock  Primitive=R1  Force=off  ForceUnits=N  Torque=off  TorqueUnits=N-m  ReferenceFrame=Absolute (INERTIAL)  ReactionSensedSide=Base  ReactionReferenceFrame=Absolute (World)  ReactionForce=off  ReactionForceUnits=N  ReactionMoment=off  ReactionMomentUnits=N-m
      settings: SourceProductName=Simscape Multibody  SourceProductBaseCode=MS
  angular velocity : mblibv1/Sensors &  Actuators/Body Sensor  Description=Mechanical Blockset  UpdateFromCAD=off  PhysicalDomain=Mechanical  PortType=blob  Muxed=on  Pose=off  Angle=on  AngleUnits=deg  ArcVelocity=on  ArcVelocityUnits=rad/s  ArcAcceleration=off  ArcAccelerationUnits=deg/s^2  CoordPosition=off  CoordPositionUnits=m  Velocity=off  VelocityUnits=m/s  Acceleration=off  AccelerationUnits=m/s^2  Quaternion=on  QuaternionDT=off  QuaternionDDT=off  QuaternionUnits=off  OutputVector=[ 3 ]  ActiveIO=on  Width=3  DialogClass=MechanicalSensorBlock  ReferenceFrame=Absolute (World)
      settings: SourceProductName=Simscape Multibody  SourceProductBaseCode=MS
  door : mblibv1/Bodies/Body  Tag=Factory generic  Description=Mechanical Blockset  LConnTagsString=CS3|CG  RConnTagsString=CS1  UpdateFromCAD=off  DialogClass=MechanicalBodyBlock  Mass=1  MassUnits=kg  InertiaUnits=kg*m^2  Inertia=eye(3)  Shape=Cylinder  ShapeDims=[1 1]  ShapeUnits=m  ShapeUse=false  Density=1  DensityUnits=kg/m^3  DensityUse=false  GraphicsMode=MACHINE_DEFAULT  BodyColorSelMode=MACHINE_DEFAULT  BodyColor=[1 0 0]  AttachedToCS=CG  CG=Left$CG$[0 0 0]$WORLD$WORLD$cm$[0 0 0]$Euler X-Y-Z$deg$WORLD$true  WorkingFrames=Left$CS3$[0 0 0]$CG$CG$cm$[0 0 0]$Euler X-Y-Z$deg$WORLD$true#Right$CS1$[17 0 0]$CG$CG$cm$[0 0 0]$Euler X-Y-Z$deg$WORLD$true  CGPos=[0 0 0]  CGRot=[0 0 0]  CS0Pos=[]  CS0Rot=[]  CS1Pos=[17 0 0]  CS1Rot=[0 0 0]  CS2Pos=[]  CS2Rot=[]  CS3Pos=[0 0 0]  CS3Rot=[0 0 0]  CS4Pos=[]  CS4Rot=[]  CS5Pos=[]  CS5Rot=[]  CS6Pos=[]  CS6Rot=[]  CS7Pos=[]  CS7Rot=[]  CS8Pos=[]  CS8Rot=[]  CS9Pos=[]  CS9Rot=[]  CS10Pos=[]  CS10Rot=[]  CS11Pos=[]  CS11Rot=[]  CS12Pos=[]  CS12Rot=[]  CS13Pos=[]  CS13Rot=[]  CS14Pos=[]  CS14Rot=[]  CS15Pos=[]  CS15Rot=[]  CS16Pos=[]  CS16Rot=[]  CS17Pos=[]  CS17Rot=[]  CS18Pos=[]  CS18Rot=[]  CS19Pos=[]  CS19Rot=[]  CS20Pos=[]  CS20Rot=[]
      settings: SourceProductName=Simscape Multibody  SourceProductBaseCode=MS
  force : Gain  Gain=-1  SaturateOnIntegerOverflow=on  OutDataTypeStr=Inherit: Same as input  ParamDataTypeStr=Inherit: Same as input
  force measurement : mblibv1/Sensors &  Actuators/Joint Sensor  Description=Mechanical Blockset  UpdateFromCAD=off  PhysicalDomain=Mechanical  PortType=blob  Muxed=on  Pose=off  Angle=on  AngleUnits=deg  ArcVelocity=off  ArcVelocityUnits=deg/s  ArcAcceleration=off  ArcAccelerationUnits=deg/s^2  CoordPosition=off  CoordPositionUnits=m  Velocity=off  VelocityUnits=m/s  Acceleration=off  AccelerationUnits=m/s^2  Quaternion=on  QuaternionDT=off  QuaternionDDT=off  QuaternionUnits=off  OutputVector=[ 3 ]  ActiveIO=on  Width=3  DialogClass=MechanicalSensorBlock  Primitive=P1  Force=off  ForceUnits=N  Torque=off  TorqueUnits=N-m  ReferenceFrame=Absolute (INERTIAL)  ReactionSensedSide=Base  ReactionReferenceFrame=Absolute (World)  ReactionForce=on  ReactionForceUnits=N  ReactionMoment=off  ReactionMomentUnits=N-m
      settings: SourceProductName=Simscape Multibody  SourceProductBaseCode=MS
  friction : Subsystem
  friction force actuation : mblibv1/Sensors &  Actuators/Joint Actuator  Description=Mechanical Blockset  UpdateFromCAD=off  PhysicalDomain=Mechanical  PortType=blob  ActuationStyle=Force  AngleUnits=deg  ArcVelocityUnits=deg/s  ArcAccelerationUnits=deg/s^2  CoordPositionUnits=m  VelocityUnits=m/s  AccelerationUnits=m/s^2  ForceUnits=N  TorqueUnits=N-m  ActiveIO=on  Width=1  DialogClass=MechanicalActuatorBlock  Primitive=P1  ReferenceFrame=Absolute (INERTIAL)
      settings: SourceProductName=Simscape Multibody  SourceProductBaseCode=MS
  main gear : mblibv1/Bodies/Body  Tag=Factory generic  Description=Mechanical Blockset  LConnTagsString=CS3|CG  RConnTagsString=CS1  UpdateFromCAD=off  DialogClass=MechanicalBodyBlock  Mass=2  MassUnits=kg  InertiaUnits=kg*m^2  Inertia=eye(3)  Shape=Cylinder  ShapeDims=[1 1]  ShapeUnits=m  ShapeUse=false  Density=1  DensityUnits=kg/m^3  DensityUse=false  GraphicsMode=MACHINE_DEFAULT  BodyColorSelMode=MACHINE_DEFAULT  BodyColor=[1 0 0]  AttachedToCS=CG  CG=Left$CG$[17 0 0]$WORLD$WORLD$cm$[0 0 0]$Euler X-Y-Z$deg$WORLD$true  WorkingFrames=Left$CS3$[0 0 0]$CG$CG$cm$[0 0 0]$Euler X-Y-Z$deg$WORLD$true#Right$CS1$[60 0 0]$CG$CG$cm$[0 0 0]$Euler X-Y-Z$deg$WORLD$true  CGPos=[17 0 0]  CGRot=[0 0 0]  CS0Pos=[]  CS0Rot=[]  CS1Pos=[60 0 0]  CS1Rot=[0 0 0]  CS2Pos=[]  CS2Rot=[]  CS3Pos=[0 0 0]  CS3Rot=[0 0 0]  CS4Pos=[]  CS4Rot=[]  CS5Pos=[]  CS5Rot=[]  CS6Pos=[]  CS6Rot=[]  CS7Pos=[]  CS7Rot=[]  CS8Pos=[]  CS8Rot=[]  CS9Pos=[]  CS9Rot=[]  CS10Pos=[]  CS10Rot=[]  CS11Pos=[]  CS11Rot=[]  CS12Pos=[]  CS12Rot=[]  CS13Pos=[]  CS13Rot=[]  CS14Pos=[]  CS14Rot=[]  CS15Pos=[]  CS15Rot=[]  CS16Pos=[]  CS16Rot=[]  CS17Pos=[]  CS17Rot=[]  CS18Pos=[]  CS18Rot=[]  CS19Pos=[]  CS19Rot=[]  CS20Pos=[]  CS20Rot=[]
      settings: SourceProductName=Simscape Multibody  SourceProductBaseCode=MS
  position & velocity measurement : mblibv1/Sensors &  Actuators/Body Sensor  Description=Mechanical Blockset  UpdateFromCAD=off  PhysicalDomain=Mechanical  PortType=blob  Muxed=on  Pose=off  Angle=on  AngleUnits=deg  ArcVelocity=off  ArcVelocityUnits=deg/s  ArcAcceleration=off  ArcAccelerationUnits=deg/s^2  CoordPosition=on  CoordPositionUnits=m  Velocity=on  VelocityUnits=m/s  Acceleration=off  AccelerationUnits=m/s^2  Quaternion=on  QuaternionDT=off  QuaternionDDT=off  QuaternionUnits=off  OutputVector=[ 3 3 ]  ActiveIO=on  Width=6  DialogClass=MechanicalSensorBlock  ReferenceFrame=Absolute (World)
      settings: SourceProductName=Simscape Multibody  SourceProductBaseCode=MS
  rotate & slide : mblibv1/Joints/Custom Joint  Tag=Factory generic  Description=Mechanical Blockset  LConnTagsString=__newl0|SA1  RConnTagsString=__newr0  UpdateFromCAD=off  NumSAPorts=1  CutJoint=off  MarkAsCut=off  Primitives=revolute_prismatic  PrimitiveProps=R1$Base$[0 0 1]$revolute#P1$Follower$[1 0 0]$prismatic  DialogClass=JointBlock  R1Axis=[0 0 1]  R2Axis=[]  R3Axis=[]  P1Axis=[1 0 0]  P2Axis=[]  P3Axis=[]  SAxis=[]
      settings: SourceProductName=Simscape Multibody  SourceProductBaseCode=MS
  torque : Gain  Gain=10000  SaturateOnIntegerOverflow=on  OutDataTypeStr=Inherit: Same as input  ParamDataTypeStr=Inherit: Same as input
  torque actuation : mblibv1/Sensors &  Actuators/Joint Actuator  Description=Mechanical Blockset  UpdateFromCAD=off  PhysicalDomain=Mechanical  PortType=blob  ActuationStyle=Force  AngleUnits=deg  ArcVelocityUnits=deg/s  ArcAccelerationUnits=deg/s^2  CoordPositionUnits=m  VelocityUnits=m/s  AccelerationUnits=m/s^2  ForceUnits=N  TorqueUnits=N-m  ActiveIO=on  Width=1  DialogClass=MechanicalActuatorBlock  Primitive=R1  ReferenceFrame=Absolute (INERTIAL)
      settings: SourceProductName=Simscape Multibody  SourceProductBaseCode=MS
  up & down : mblibv1/Joints/Prismatic  Tag=Factory generic  Description=Mechanical Blockset  LConnTagsString=__newl0|SA1  RConnTagsString=__newr0|SA1  UpdateFromCAD=off  NumSAPorts=2  CutJoint=on  MarkAsCut=off  Primitives=prismatic  PrimitiveProps=P1$WORLD$[0 1 0]$prismatic  DialogClass=JointBlock  P1Axis=[0 1 0]
      settings: SourceProductName=Simscape Multibody  SourceProductBaseCode=MS
  window : mblibv1/Bodies/Body  Tag=Factory generic  Description=Mechanical Blockset  LConnTagsString=CS1  RConnTagsString=CS2|CS3  UpdateFromCAD=off  DialogClass=MechanicalBodyBlock  Mass=5  MassUnits=kg  InertiaUnits=kg*m^2  Inertia=eye(3)  Shape=Cylinder  ShapeDims=[1 1]  ShapeUnits=m  ShapeUse=false  Density=1  DensityUnits=kg/m^3  DensityUse=false  GraphicsMode=MACHINE_DEFAULT  BodyColorSelMode=MACHINE_DEFAULT  BodyColor=[1 0 0]  AttachedToCS=CG  CG=Left$CG$[10 0 0]$WORLD$WORLD$cm$[0 0 0]$Euler X-Y-Z$deg$WORLD$false  WorkingFrames=Left$CS1$[0 0 0]$CG$CG$cm$[0 0 0]$Euler X-Y-Z$deg$WORLD$true#Right$CS2$[0 0 0]$CG$CG$cm$[0 0 0]$Euler X-Y-Z$deg$WORLD$true#Right$CS3$[-15 0 0]$CG$CG$cm$[0 0 0]$Euler X-Y-Z$deg$WORLD$true  CGPos=[10 0 0]  CGRot=[0 0 0]  CS0Pos=[]  CS0Rot=[]  CS1Pos=[0 0 0]  CS1Rot=[0 0 0]  CS2Pos=[0 0 0]  CS2Rot=[0 0 0]  CS3Pos=[-15 0 0]  CS3Rot=[0 0 0]  CS4Pos=[]  CS4Rot=[]  CS5Pos=[]  CS5Rot=[]  CS6Pos=[]  CS6Rot=[]  CS7Pos=[]  CS7Rot=[]  CS8Pos=[]  CS8Rot=[]  CS9Pos=[]  CS9Rot=[]  CS10Pos=[]  CS10Rot=[]  CS11Pos=[]  CS11Rot=[]  CS12Pos=[]  CS12Rot=[]  CS13Pos=[]  CS13Rot=[]  CS14Pos=[]  CS14Rot=[]  CS15Pos=[]  CS15Rot=[]  CS16Pos=[]  CS16Rot=[]  CS17Pos=[]  CS17Rot=[]  CS18Pos=[]  CS18Rot=[]  CS19Pos=[]  CS19Rot=[]  CS20Pos=[]  CS20Rot=[]
      settings: SourceProductName=Simscape Multibody  SourceProductBaseCode=MS
  worm : mblibv1/Bodies/Body  Tag=Factory generic  Description=Mechanical Blockset  LConnTagsString=CS3|CS4  RConnTagsString=CG  UpdateFromCAD=off  DialogClass=MechanicalBodyBlock  Mass=0.5  MassUnits=kg  InertiaUnits=kg*m^2  Inertia=eye(3)  Shape=Cylinder  ShapeDims=[1 1]  ShapeUnits=m  ShapeUse=false  Density=1  DensityUnits=kg/m^3  DensityUse=false  GraphicsMode=MACHINE_DEFAULT  BodyColorSelMode=MACHINE_DEFAULT  BodyColor=[1 0 0]  AttachedToCS=CG  CG=Right$CG$[0 0 0]$WORLD$WORLD$cm$[0 0 0]$Euler X-Y-Z$deg$WORLD$true  WorkingFrames=Left$CS3$[0 0 0]$CG$CG$cm$[0 0 0]$Euler X-Y-Z$deg$WORLD$true#Left$CS4$[0 0 0]$CG$CG$cm$[0 0 0]$Euler X-Y-Z$deg$WORLD$true  CGPos=[0 0 0]  CGRot=[0 0 0]  CS0Pos=[]  CS0Rot=[]  CS1Pos=[]  CS1Rot=[]  CS2Pos=[]  CS2Rot=[]  CS3Pos=[0 0 0]  CS3Rot=[0 0 0]  CS4Pos=[0 0 0]  CS4Rot=[0 0 0]  CS5Pos=[]  CS5Rot=[]  CS6Pos=[]  CS6Rot=[]  CS7Pos=[]  CS7Rot=[]  CS8Pos=[]  CS8Rot=[]  CS9Pos=[]  CS9Rot=[]  CS10Pos=[]  CS10Rot=[]  CS11Pos=[]  CS11Rot=[]  CS12Pos=[]  CS12Rot=[]  CS13Pos=[]  CS13Rot=[]  CS14Pos=[]  CS14Rot=[]  CS15Pos=[]  CS15Rot=[]  CS16Pos=[]  CS16Rot=[]  CS17Pos=[]  CS17Rot=[]  CS18Pos=[]  CS18Rot=[]  CS19Pos=[]  CS19Rot=[]  CS20Pos=[]  CS20Rot=[]
      settings: SourceProductName=Simscape Multibody  SourceProductBaseCode=MS
  worm gear : mblibv1/Constraints &  Drivers/Gear Constraint  Tag=Factory generic  Description=Mechanical Blockset  LConnTagsString=__newl0  RConnTagsString=__newr0  UpdateFromCAD=off  DialogClass=GearConstraint  NumSAPorts=0  BaseRadius=2  BaseRadiusUnits=cm  FollowerRadius=15  FollowerRadiusUnits=cm
      settings: SourceProductName=Simscape Multibody  SourceProductBaseCode=MS
  F,d,v : Outport
  ti : Outport  Port=2
  q : Outport  Port=3
  wires:
  angle measurement/1 -> q/1
  Mux/1 -> F,d,v/1
  force measurement/1 -> Mux/1
  position & velocity measurement/1 -> Mux/2, Demux1/1
  Demux1/2 -> friction/1(position)
  Demux1/5 -> friction/2(velocity)
  torque/1 -> ti/1, torque actuation/1
  Sum2/1 -> torque/1
  angular velocity/1 -> Demux2/1
  Demux2/3 -> Sum2/1
  wi/1 -> Sum2/2
  Fx/1 -> Sum1/2
  friction/1(torque) -> Sum1/1
  Sum1/1 -> force/1
  force/1 -> friction force actuation/1
  Demux1/6 -> Terminator1/1
  Demux1/4 -> Terminator2/1
  Demux1/3 -> Terminator3/1
  Demux1/1 -> Terminator4/1
  Demux2/1 -> Terminator5/1
  Demux2/2 -> Terminator6/1
  connections:
  rotate & slide/LConn2 -- angle measurement/LConn1
  force measurement/LConn1 -- up & down/RConn2
  friction force actuation/RConn1 -- up & down/LConn2
  Revolute8/RConn1 -- worm/LConn2
  worm/LConn1 -- worm gear/LConn1
  door/RConn1 -- Revolute1/LConn1
  Revolute1/RConn1 -- main gear/LConn2
  worm gear/RConn1 -- main gear/LConn1
  door/LConn1 -- Revolute6/RConn1
  torque actuation/RConn1 -- Revolute8/LConn2
  door/LConn2 -- Revolute8/LConn1
  main gear/RConn1 -- rotate & slide/LConn1
  rotate & slide/RConn1 -- window/LConn1
  window/RConn2 -- position & velocity measurement/LConn1
  GND/RConn1 -- up & down/LConn1
  up & down/RConn1 -- window/RConn1
  worm/RConn1 -- angular velocity/LConn1
  Revolute6/LConn1 -- GND2/RConn1
  GND/LConn1 -- Machine Environment/RConn1

== system powerwindow03/window_system/plant/window/Atomic Subsystem ==

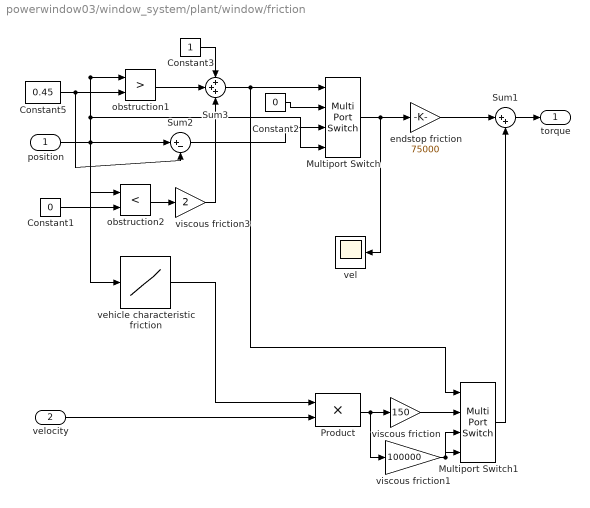
== system powerwindow03/window_system/plant/window/friction ==
  position : Inport
  velocity : Inport  Port=2
  Constant1 : Constant  Value=0
  Constant2 : Constant  Value=0
  Constant3 : Constant
  Constant5 : Constant  Value=0.45
  Multiport Switch : MultiPortSwitch  InputSameDT=on
  Multiport Switch1 : MultiPortSwitch  InputSameDT=on
  Product : Product  SaturateOnIntegerOverflow=on  InputSameDT=on  OutDataTypeStr=Inherit: Same as first input
  Sum1 : Sum  Inputs=|++  SaturateOnIntegerOverflow=on  InputSameDT=on  OutDataTypeStr=Inherit: Same as first input
  Sum2 : Sum  Inputs=|+-  SaturateOnIntegerOverflow=on  InputSameDT=on  OutDataTypeStr=Inherit: Same as first input
  Sum3 : Sum  Inputs=+++  SaturateOnIntegerOverflow=on  InputSameDT=on  OutDataTypeStr=Inherit: Same as first input
  endstop friction : Gain  Gain=75000  SaturateOnIntegerOverflow=on  OutDataTypeStr=Inherit: Same as input  ParamDataTypeStr=Inherit: Same as input
  obstruction1 : RelationalOperator  Operator=>  RndMeth=Nearest  InputSameDT=on
  obstruction2 : RelationalOperator  Operator=<  RndMeth=Nearest  InputSameDT=on
  vehicle characteristic friction : Lookup_n-D  NumberOfTableDimensions=1  BreakpointsForDimension1=[0 2.5 10 11.5 14 24 30 31 35 47 50]  Table=[1.15 1.2 1.05 1.1 1.05 1 1.1 1 0.95 0.9 0.95]  SaturateOnIntegerOverflow=on  InputSameDT=on
  vel : Scope
  viscous friction3 : Gain  Gain=2  SaturateOnIntegerOverflow=on  OutDataTypeStr=Inherit: Same as input  ParamDataTypeStr=Inherit: Same as input
  viscous friction : Gain  Gain=150  SaturateOnIntegerOverflow=on  OutDataTypeStr=Inherit: Same as input  ParamDataTypeStr=Inherit: Same as input
  viscous friction1 : Gain  Gain=100000  SaturateOnIntegerOverflow=on  OutDataTypeStr=Inherit: Same as input  ParamDataTypeStr=Inherit: Same as input
  torque : Outport
  wires:
  Sum1/1 -> torque/1
  velocity/1 -> Product/2
  position/1 -> obstruction1/1, obstruction2/1, Multiport Switch/4, Sum2/1, vehicle characteristic friction/1
  Constant5/1 -> obstruction1/2, Sum2/2
  Constant1/1 -> obstruction2/2
  endstop friction/1 -> Sum1/1
  Constant2/1 -> Multiport Switch/2
  Sum2/1 -> Multiport Switch/3
  obstruction2/1 -> viscous friction3/1
  obstruction1/1 -> Sum3/2
  viscous friction3/1 -> Sum3/3
  Constant3/1 -> Sum3/1
  Sum3/1 -> Multiport Switch/1, Multiport Switch1/1
  Multiport Switch/1 -> endstop friction/1, vel/1
  Product/1 -> viscous friction/1, viscous friction1/1
  vehicle characteristic friction/1 -> Product/1
  viscous friction/1 -> Multiport Switch1/2
  Multiport Switch1/1 -> Sum1/2
  viscous friction1/1 -> Multiport Switch1/3, Multiport Switch1/4
